simulink subsystem "GS3DX_KDS_Gimbal"  (R2025b)
settings: Solver=VariableStepAuto  StartTime=0.0  StopTime=10.0  RelTol=1e-3
model mask{StartPositionX=0, StartPositionY=0, StartPositionZ=0, StartVelocityX=0, StartVelocityY=0, StartVelocityZ=0, DampeningX=0, DampeningY=0, DampeningZ=0, RxPositionTargetPriority=None, RyPositionTargetPriority=None, RzPositionTargetPriority=None, RxVelocityTargetPriority=None, RyVelocityTargetPriority=None, RzVelocityTargetPriority=None}
  mask prompts: StartPositionX "Start Position X (deg)"; StartPositionY "Start Position Y (deg)"; StartPositionZ "Start Position Z (deg)"; StartVelocityX "Start Velocity X (deg/s)"; StartVelocityY "Start Velocity Y (deg/s)"; StartVelocityZ "Start Velocity Z (deg/s)"; DampeningX "Dampening X (Nm/deg/s)"; DampeningY "Dampening Y (Nm/deg/s)"; DampeningZ "Dampening Z (Nm/deg/s)"; RxPositionTargetPriority "Position Target Priority X"; RyPositionTargetPriority "Position Target Priority Y"; RzPositionTargetPriority "Position Target Priority Z"; RxVelocityTargetPriority "Velocity Target Priority X"; RyVelocityTargetPriority "Velocity Target Priority Y"; RzVelocityTargetPriority "Velocity Target Priority Z"
undefined symbols (not defined in the file): DampeningGlobalGain, LocalDampeningEnable
libraries: nesl_utility x24, sm_lib x3
settings Model: Creator=diete  LastModifiedBy=diete

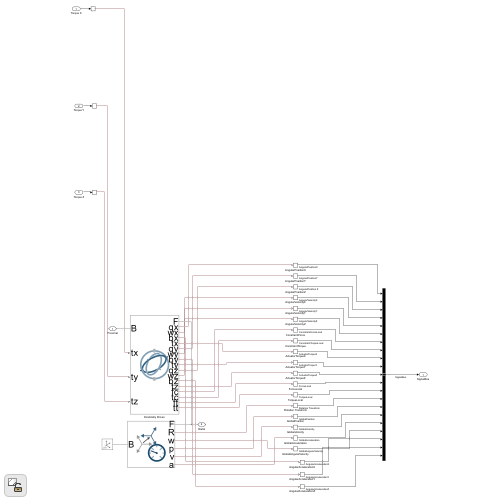
[thumbnail: Simulink's stored preview of the top-level diagram]
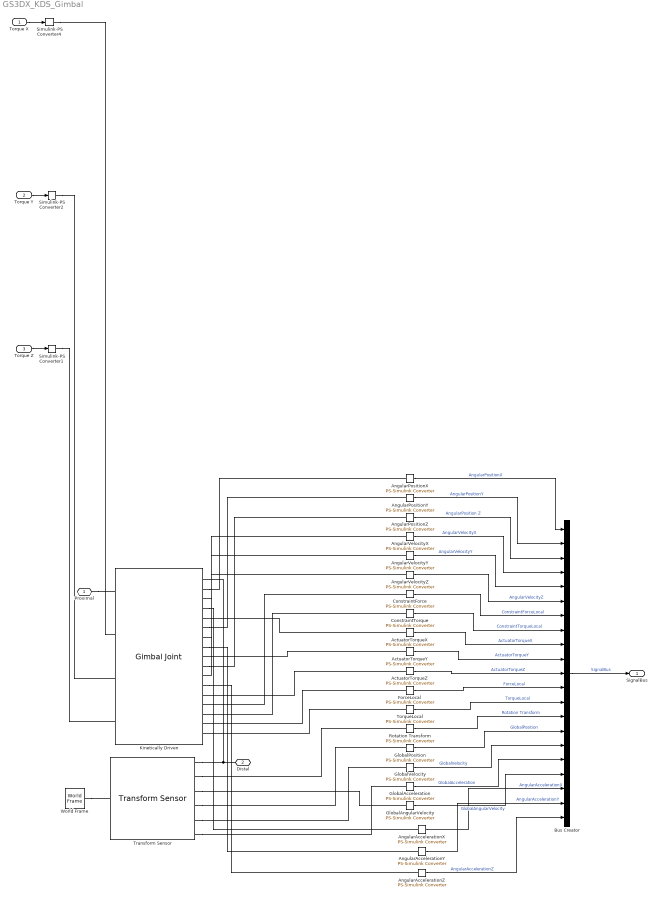
== system GS3DX_KDS_Gimbal ==
  Torque X : Inport
  Torque Y : Inport  Port=2
  Torque Z : Inport  Port=3
  ActuatorTorqueX : nesl_utility/PS-Simulink Converter  PhysicalDomain=network_engine_domain  SubClassName=ps_output  LeftPortType=input  RightPortType=output  PseudoPeriodic=off  Frequencies=[]  VectorFormat=1-D array  Unit=inherit  AffineConversion=off
  ActuatorTorqueY : nesl_utility/PS-Simulink Converter  PhysicalDomain=network_engine_domain  SubClassName=ps_output  LeftPortType=input  RightPortType=output  PseudoPeriodic=off  Frequencies=[]  VectorFormat=1-D array  Unit=inherit  AffineConversion=off
  ActuatorTorqueZ : nesl_utility/PS-Simulink Converter  PhysicalDomain=network_engine_domain  SubClassName=ps_output  LeftPortType=input  RightPortType=output  PseudoPeriodic=off  Frequencies=[]  VectorFormat=1-D array  Unit=inherit  AffineConversion=off
  AngularAccelerationX : nesl_utility/PS-Simulink Converter  PhysicalDomain=network_engine_domain  SubClassName=ps_output  LeftPortType=input  RightPortType=output  PseudoPeriodic=off  Frequencies=[]  VectorFormat=1-D array  Unit=deg/s^2  AffineConversion=off
  AngularAccelerationY : nesl_utility/PS-Simulink Converter  PhysicalDomain=network_engine_domain  SubClassName=ps_output  LeftPortType=input  RightPortType=output  PseudoPeriodic=off  Frequencies=[]  VectorFormat=1-D array  Unit=deg/s^2  AffineConversion=off
  AngularAccelerationZ : nesl_utility/PS-Simulink Converter  PhysicalDomain=network_engine_domain  SubClassName=ps_output  LeftPortType=input  RightPortType=output  PseudoPeriodic=off  Frequencies=[]  VectorFormat=1-D array  Unit=deg/s^2  AffineConversion=off
  AngularPositionX : nesl_utility/PS-Simulink Converter  PhysicalDomain=network_engine_domain  SubClassName=ps_output  LeftPortType=input  RightPortType=output  PseudoPeriodic=off  Frequencies=[]  VectorFormat=1-D array  Unit=deg  AffineConversion=off
  AngularPositionY : nesl_utility/PS-Simulink Converter  PhysicalDomain=network_engine_domain  SubClassName=ps_output  LeftPortType=input  RightPortType=output  PseudoPeriodic=off  Frequencies=[]  VectorFormat=1-D array  Unit=deg  AffineConversion=off
  AngularPositionZ : nesl_utility/PS-Simulink Converter  PhysicalDomain=network_engine_domain  SubClassName=ps_output  LeftPortType=input  RightPortType=output  PseudoPeriodic=off  Frequencies=[]  VectorFormat=1-D array  Unit=deg  AffineConversion=off
  AngularVelocityX : nesl_utility/PS-Simulink Converter  PhysicalDomain=network_engine_domain  SubClassName=ps_output  LeftPortType=input  RightPortType=output  PseudoPeriodic=off  Frequencies=[]  VectorFormat=1-D array  Unit=deg/s  AffineConversion=off
  AngularVelocityY : nesl_utility/PS-Simulink Converter  PhysicalDomain=network_engine_domain  SubClassName=ps_output  LeftPortType=input  RightPortType=output  PseudoPeriodic=off  Frequencies=[]  VectorFormat=1-D array  Unit=deg/s  AffineConversion=off
  AngularVelocityZ : nesl_utility/PS-Simulink Converter  PhysicalDomain=network_engine_domain  SubClassName=ps_output  LeftPortType=input  RightPortType=output  PseudoPeriodic=off  Frequencies=[]  VectorFormat=1-D array  Unit=deg/s  AffineConversion=off
  Bus Creator : BusCreator  Inputs=21
  ConstraintForce : nesl_utility/PS-Simulink Converter  PhysicalDomain=network_engine_domain  SubClassName=ps_output  LeftPortType=input  RightPortType=output  PseudoPeriodic=off  Frequencies=[]  VectorFormat=1-D array  Unit=inherit  AffineConversion=off
  ConstraintTorque : nesl_utility/PS-Simulink Converter  PhysicalDomain=network_engine_domain  SubClassName=ps_output  LeftPortType=input  RightPortType=output  PseudoPeriodic=off  Frequencies=[]  VectorFormat=1-D array  Unit=inherit  AffineConversion=off
  ForceLocal : nesl_utility/PS-Simulink Converter  PhysicalDomain=network_engine_domain  SubClassName=ps_output  LeftPortType=input  RightPortType=output  PseudoPeriodic=off  Frequencies=[]  VectorFormat=1-D array  Unit=inherit  AffineConversion=off
  GlobalAcceleration : nesl_utility/PS-Simulink Converter  PhysicalDomain=network_engine_domain  SubClassName=ps_output  LeftPortType=input  RightPortType=output  PseudoPeriodic=off  Frequencies=[]  VectorFormat=1-D array  Unit=inherit  AffineConversion=off
  GlobalAngularVelocity : nesl_utility/PS-Simulink Converter  PhysicalDomain=network_engine_domain  SubClassName=ps_output  LeftPortType=input  RightPortType=output  PseudoPeriodic=off  Frequencies=[]  VectorFormat=1-D array  Unit=deg/s  AffineConversion=off
  GlobalPosition : nesl_utility/PS-Simulink Converter  PhysicalDomain=network_engine_domain  SubClassName=ps_output  LeftPortType=input  RightPortType=output  PseudoPeriodic=off  Frequencies=[]  VectorFormat=1-D array  Unit=inherit  AffineConversion=off
  GlobalVelocity : nesl_utility/PS-Simulink Converter  PhysicalDomain=network_engine_domain  SubClassName=ps_output  LeftPortType=input  RightPortType=output  PseudoPeriodic=off  Frequencies=[]  VectorFormat=1-D array  Unit=inherit  AffineConversion=off
  Kinetically Driven : sm_lib/Joints/Gimbal Joint  JointMode=Normal  CompositeWrenchDir=BaseOnFollower  CompositeWrenchFrame=FollowerFrame  SenseConstraintForce=on  SenseConstraintTorque=on  SenseTotalForce=on  SenseTotalTorque=on  RxPositionTargetSpecify=off  RxPositionTargetPriority=High  RxPositionTargetValue=StartPositionX  RxPositionTargetValueUnits=deg  RxVelocityTargetSpecify=off  RxVelocityTargetPriority=High  RxVelocityTargetValue=StartVelocityX  RxVelocityTargetValueUnits=deg/s  RxEquilibriumPosition=0  RxEquilibriumPositionUnits=deg  RxSpringStiffness=0  RxSpringStiffnessUnits=N*m/deg  RxDampingCoefficient=DampeningX*LocalDampeningEnable*DampeningGlobalGain  RxDampingCoefficientUnits=N*m/(deg/s)  RxLowerLimitSpecify=off  RxLowerLimitBound=-80  RxLowerLimitBoundUnits=deg  RxLowerLimitStiffness=100  RxLowerLimitStiffnessUnits=N*m/deg  RxLowerLimitDamping=10  RxLowerLimitDampingUnits=N*m/(deg/s)  RxLowerLimitTransitionRegionWidth=0.1  RxLowerLimitTransitionRegionWidthUnits=deg  RxUpperLimitSpecify=off  RxUpperLimitBound=80  RxUpperLimitBoundUnits=deg  RxUpperLimitStiffness=100  RxUpperLimitStiffnessUnits=N*m/deg  RxUpperLimitDamping=10  RxUpperLimitDampingUnits=N*m/(deg/s)  RxUpperLimitTransitionRegionWidth=0.1  RxUpperLimitTransitionRegionWidthUnits=deg  RxTorqueActuationMode=InputTorque  RxMotionActuationMode=ComputedMotion  RxSensePosition=on  RxSenseVelocity=on  RxSenseAcceleration=on  RxSenseTorqueForce=on  RxSenseLowerLimitTorqueForce=off  RxSenseUpperLimitTorqueForce=off  RyPositionTargetSpecify=off  RyPositionTargetPriority=High  RyPositionTargetValue=StartPositionY  RyPositionTargetValueUnits=deg  RyVelocityTargetSpecify=off  RyVelocityTargetPriority=High  RyVelocityTargetValue=StartVelocityY  RyVelocityTargetValueUnits=deg/s  RyEquilibriumPosition=0  RyEquilibriumPositionUnits=deg  RySpringStiffness=0  RySpringStiffnessUnits=N*m/deg  RyDampingCoefficient=DampeningY*LocalDampeningEnable*DampeningGlobalGain  RyDampingCoefficientUnits=N*m/(deg/s)  RyLowerLimitSpecify=off  RyLowerLimitBound=-80  RyLowerLimitBoundUnits=deg  RyLowerLimitStiffness=100  RyLowerLimitStiffnessUnits=N*m/deg  RyLowerLimitDamping=10  RyLowerLimitDampingUnits=N*m/(deg/s)  RyLowerLimitTransitionRegionWidth=0.1  RyLowerLimitTransitionRegionWidthUnits=deg  RyUpperLimitSpecify=off  RyUpperLimitBound=80  RyUpperLimitBoundUnits=deg  RyUpperLimitStiffness=100  RyUpperLimitStiffnessUnits=N*m/deg  RyUpperLimitDamping=10  RyUpperLimitDampingUnits=N*m/(deg/s)  RyUpperLimitTransitionRegionWidth=0.1  RyUpperLimitTransitionRegionWidthUnits=deg  RyTorqueActuationMode=InputTorque  RyMotionActuationMode=ComputedMotion  RySensePosition=on  RySenseVelocity=on  RySenseAcceleration=on  RySenseTorqueForce=on  RySenseLowerLimitTorqueForce=off  RySenseUpperLimitTorqueForce=off  RzPositionTargetSpecify=off  RzPositionTargetPriority=High  RzPositionTargetValue=StartPositionZ  RzPositionTargetValueUnits=deg  RzVelocityTargetSpecify=off  RzVelocityTargetPriority=High  RzVelocityTargetValue=StartVelocityZ  RzVelocityTargetValueUnits=deg/s  RzEquilibriumPosition=0  RzEquilibriumPositionUnits=deg  RzSpringStiffness=0  RzSpringStiffnessUnits=N*m/deg  RzDampingCoefficient=DampeningZ*LocalDampeningEnable*DampeningGlobalGain  RzDampingCoefficientUnits=N*m/(deg/s)  RzLowerLimitSpecify=off  RzLowerLimitBound=-180  RzLowerLimitBoundUnits=deg  RzLowerLimitStiffness=100  RzLowerLimitStiffnessUnits=N*m/deg  RzLowerLimitDamping=10  RzLowerLimitDampingUnits=N*m/(deg/s)  RzLowerLimitTransitionRegionWidth=0.1  RzLowerLimitTransitionRegionWidthUnits=deg  RzUpperLimitSpecify=off  RzUpperLimitBound=-95  RzUpperLimitBoundUnits=deg  RzUpperLimitStiffness=100  RzUpperLimitStiffnessUnits=N*m/deg  RzUpperLimitDamping=10  RzUpperLimitDampingUnits=N*m/(deg/s)  RzUpperLimitTransitionRegionWidth=0.1  RzUpperLimitTransitionRegionWidthUnits=deg  RzTorqueActuationMode=InputTorque  RzMotionActuationMode=ComputedMotion  RzSensePosition=on  RzSenseVelocity=on  RzSenseAcceleration=on  RzSenseTorqueForce=on  RzSenseLowerLimitTorqueForce=off  RzSenseUpperLimitTorqueForce=off
  Rotation Transform : nesl_utility/PS-Simulink Converter  PhysicalDomain=network_engine_domain  SubClassName=ps_output  LeftPortType=input  RightPortType=output  PseudoPeriodic=off  Frequencies=[]  VectorFormat=1-D array  Unit=inherit  AffineConversion=off
  Simulink-PS Converter1 : nesl_utility/Simulink-PS Converter  PhysicalDomain=network_engine_domain  SubClassName=ps_input  LeftPortType=input  RightPortType=output  PseudoPeriodic=off  Frequencies=[]  NoiseDistribution=none  NoiseParameters=[]  Unit=1  AffineConversion=off  FilteringAndDerivatives=provide  SimscapeFilterOrder=1  InputFilterTimeConstant=0.001  UdotUserProvided=0
  Simulink-PS Converter2 : nesl_utility/Simulink-PS Converter  PhysicalDomain=network_engine_domain  SubClassName=ps_input  LeftPortType=input  RightPortType=output  PseudoPeriodic=off  Frequencies=[]  NoiseDistribution=none  NoiseParameters=[]  Unit=1  AffineConversion=off  FilteringAndDerivatives=provide  SimscapeFilterOrder=1  InputFilterTimeConstant=0.001  UdotUserProvided=0
  Simulink-PS Converter4 : nesl_utility/Simulink-PS Converter  PhysicalDomain=network_engine_domain  SubClassName=ps_input  LeftPortType=input  RightPortType=output  PseudoPeriodic=off  Frequencies=[]  NoiseDistribution=none  NoiseParameters=[]  Unit=1  AffineConversion=off  FilteringAndDerivatives=provide  SimscapeFilterOrder=1  InputFilterTimeConstant=0.001  UdotUserProvided=0
  TorqueLocal : nesl_utility/PS-Simulink Converter  PhysicalDomain=network_engine_domain  SubClassName=ps_output  LeftPortType=input  RightPortType=output  PseudoPeriodic=off  Frequencies=[]  VectorFormat=1-D array  Unit=inherit  AffineConversion=off
  Transform Sensor : sm_lib/Frames and Transforms/Transform Sensor  MeasurementFrame=World  RotationSequence=XYX  SenseAngle=off  SenseAxis=off  SenseQ=off  SenseR=on  SenseRotationSequence=off  SenseOmegaX=off  SenseOmegaY=off  SenseOmegaZ=off  SenseOmega=on  SenseQDot=off  SenseRDot=off  SenseRotationSequenceDot=off  SenseAlphaX=off  SenseAlphaY=off  SenseAlphaZ=off  SenseAlpha=off  SenseQDDot=off  SenseRDDot=off  SenseX=off  SenseY=off  SenseZ=off  SenseXYZ=on  SenseRad=off  SenseAzim=off  SenseDist=off  SenseInc=off  SenseXDot=off  SenseYDot=off  SenseZDot=off  SenseXYZDot=on  SenseRadDot=off  SenseAzimDot=off  SenseDistDot=off  SenseIncDot=off  SenseXDDot=off  SenseYDDot=off  SenseZDDot=off  SenseXYZDDot=on  SenseRadDDot=off  SenseAzimDDot=off  SenseDistDDot=off  SenseIncDDot=off
  World Frame : sm_lib/Frames and Transforms/World Frame
  Proximal : PMIOPort  Side=Left
  Distal : PMIOPort  Port=2  Side=Right
  SignalBus : Outport
  wires:
  Rotation Transform/1 -> Bus Creator/14  "Rotation Transform"
  ActuatorTorqueY/1 -> Bus Creator/10  "ActuatorTorqueY"
  ForceLocal/1 -> Bus Creator/12  "ForceLocal"
  ConstraintTorque/1 -> Bus Creator/8  "ConstraintTorqueLocal"
  GlobalAcceleration/1 -> Bus Creator/17  "GlobalAcceleration"
  GlobalAngularVelocity/1 -> Bus Creator/18  "GlobalAngularVelocity"
  Torque X/1 -> Simulink-PS Converter4/1
  ConstraintForce/1 -> Bus Creator/7  "ConstraintForceLocal"
  AngularVelocityY/1 -> Bus Creator/5  "AngularVelocityY"
  AngularPositionY/1 -> Bus Creator/2  "AngularPositionY"
  Torque Y/1 -> Simulink-PS Converter2/1
  ActuatorTorqueX/1 -> Bus Creator/9  "ActuatorTorqueX"
  AngularPositionX/1 -> Bus Creator/1  "AngularPositionX"
  TorqueLocal/1 -> Bus Creator/13  "TorqueLocal"
  GlobalVelocity/1 -> Bus Creator/16  "GlobalVelocity"
  GlobalPosition/1 -> Bus Creator/15  "GlobalPosition"
  Bus Creator/1 -> SignalBus/1  "SignalBus"
  AngularVelocityX/1 -> Bus Creator/4  "AngularVelocityX"
  Torque Z/1 -> Simulink-PS Converter1/1
  ActuatorTorqueZ/1 -> Bus Creator/11  "ActuatorTorqueZ"
  AngularVelocityZ/1 -> Bus Creator/6  "AngularVelocityZ"
  AngularPositionZ/1 -> Bus Creator/3  "AngularPosition Z"
  AngularAccelerationX/1 -> Bus Creator/19  "AngularAccelerationX"
  AngularAccelerationY/1 -> Bus Creator/20  "AngularAccelerationY"
  AngularAccelerationZ/1 -> Bus Creator/21  "AngularAccelerationZ"
  connections:
  Transform Sensor/RConn1 -- Distal/RConn1 -- Kinetically Driven/RConn1
  Transform Sensor/RConn4 -- GlobalPosition/LConn1
  Proximal/RConn1 -- Kinetically Driven/LConn1
  Transform Sensor/RConn2 -- Rotation Transform/LConn1
  Transform Sensor/RConn3 -- GlobalAngularVelocity/LConn1
  Transform Sensor/RConn6 -- GlobalAcceleration/LConn1
  Transform Sensor/RConn5 -- GlobalVelocity/LConn1
  World Frame/RConn1 -- Transform Sensor/LConn1
  TorqueLocal/LConn1 -- Kinetically Driven/RConn17
  ForceLocal/LConn1 -- Kinetically Driven/RConn16
  ActuatorTorqueZ/LConn1 -- Kinetically Driven/RConn13
  ActuatorTorqueY/LConn1 -- Kinetically Driven/RConn9
  ActuatorTorqueX/LConn1 -- Kinetically Driven/RConn5
  ConstraintTorque/LConn1 -- Kinetically Driven/RConn15
  ConstraintForce/LConn1 -- Kinetically Driven/RConn14
  Kinetically Driven/RConn2 -- AngularPositionX/LConn1
  Kinetically Driven/RConn6 -- AngularPositionY/LConn1
  Kinetically Driven/RConn10 -- AngularPositionZ/LConn1
  Kinetically Driven/RConn4 -- AngularAccelerationX/LConn1
  Kinetically Driven/RConn8 -- AngularAccelerationY/LConn1
  Kinetically Driven/RConn12 -- AngularAccelerationZ/LConn1
  AngularVelocityX/LConn1 -- Kinetically Driven/RConn3
  AngularVelocityY/LConn1 -- Kinetically Driven/RConn7
  AngularVelocityZ/LConn1 -- Kinetically Driven/RConn11
  Simulink-PS Converter2/RConn1 -- Kinetically Driven/LConn3
  Simulink-PS Converter4/RConn1 -- Kinetically Driven/LConn2
  Simulink-PS Converter1/RConn1 -- Kinetically Driven/LConn4
